simulink model "single_form_optimization"  (R2020a)
settings: Solver=VariableStepAuto  StartTime=0.0  StopTime=totalTime  RelTol=1e-3
undefined symbols (not defined in the file or in its folder): pw, totalTime
settings Model: OrderedModelArguments=off  Creator=wuyua  LastModifiedBy=wuyua

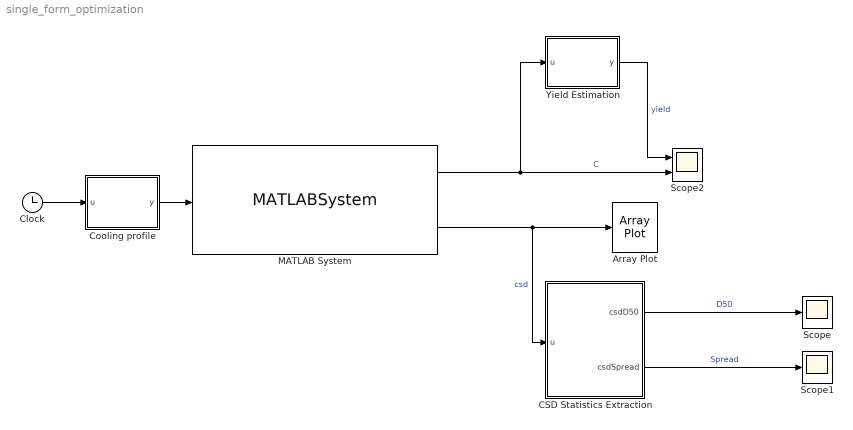
== system single_form_optimization ==
  Array Plot : ArrayPlot
  CSD Statistics Extraction : MATLAB Function  TreatAsAtomicUnit=on
  Clock : Clock
  Cooling profile : MATLAB Function  TreatAsAtomicUnit=on
  MATLAB System : MATLABSystem  System=solver_system  sampleTimeSecond=sampleTime  cfl=cfl  solverObj=s  ic=ic  SimulateUsing=Interpreted execution
      mask Type: solver_system
      mask Display:
      | disp('solver_system');
      | port_label('input',1,'u');
      | port_label('output',1,'c');
      | port_label('output',2,'csd1');
  Scope : Scope
  Scope1 : Scope
  Scope2 : Scope  NumInputPorts=2
  Yield Estimation : MATLAB Function  TreatAsAtomicUnit=on
  wires:
  Cooling profile/1(y) -> MATLAB System/1
  MATLAB System/1 -> Yield Estimation/1(u), Scope2/2  "C"
  MATLAB System/2 -> CSD Statistics Extraction/1(u), Array Plot/1  "csd"
  CSD Statistics Extraction/1(csdD50) -> Scope/1  "D50"
  CSD Statistics Extraction/2(csdSpread) -> Scope1/1  "Spread"
  Clock/1 -> Cooling profile/1(u)
  Yield Estimation/1(y) -> Scope2/1  "yield"

== matlab function single_form_optimization/CSD Statistics Extraction ==
  data: u input; csdD50 output size=1; csdSpread output size=1
function [csdD50, csdSpread] = fcn(u)
cumulative = cumtrapz(u);
normalized = cumulative/cumulative(end);
normalized = normalized(normalized<1.0);
if numel(normalized) <= 2
    csdD50 = 0;
    csdSpread = NaN;
    return;
end
g = linspace(0, numel(normalized), numel(normalized));

csdD50 = interp1(normalized, g, 0.5);
y = interp1(normalized, g, [0.9 0.1]);

csdSpread = y(1)-y(2);

== matlab function single_form_optimization/Yield Estimation ==
  data: u input; y output; initConc parameter
function y = fcn(u, initConc)
solute = initConc;
prodSolid = initConc - u;

y = prodSolid/solute;

== matlab function single_form_optimization/Cooling profile ==
  data: u input; y output; pw parameter; totalTime parameter
function y = fcn(u, pw, totalTime)

y = (1-(u/totalTime).^pw) * 40 + 10;
